simulink model "Manoel_05"  (R2018a)
settings: Solver=VariableStepAuto  StartTime=0.0  StopTime=10.0  RelTol=1e-3
values from neighbouring files (symbols this model uses):
  A = [-4.5 0; 1 -0.2]    [manoel_outubro2.m]    (also in pre6_teste.m; pre_lab5.m; pre_lab6.m; pre_pedro.m = [-5.5 0; 1 -8.40])
  atraso = stt    [manoel_outubro2.m]    (also in naao_roda.m = infor.SettlingTime; pre6_teste.m = infor.SettlingTime; pre_lab3.m = infor.SettlingTime; pre_lab3_lab.m = infor.SettlingTime)
  B = [21.6; 0]    [manoel_outubro2.m]    (also in pre6_teste.m; pre_lab5.m = [18; 0]; pre_lab6.m = [b0; 0]; pre_pedro.m = [462; 0])
  ganho = 0.01027*infor.SettlingMax    [manoel_outubro2.m]    (also in naao_roda.m; pre6_teste.m; pre_lab3.m; pre_lab3_lab.m)
  K = place(Ad, Bd, polos)    [pre6_teste.m]    (also in pre_lab5.m; pre_pedro.m = place(F, H, Dinamica))
  Kpf = 1.0436    [pre_lab3.m]    (also in pre_lab3_lab.m; pre_lab4.m; pre_pedro.m = 1/dcgain(EE))
  R0 = round(r0,1)    [naao_roda.m]    (also in pre6_teste.m; pre_lab3.m; pre_lab3_lab.m; pre_lab4.m)
  T0 = round(t0,3)    [naao_roda.m]    (also in pre6_teste.m = 0.063; pre_lab3.m; pre_lab3_2.m = 0.0640576; pre_lab3_lab.m)
undefined symbols (not defined in the file or in its folder): Ad, Bd
settings Model: Creator=joaovitor  LastModifiedBy=joaovitor

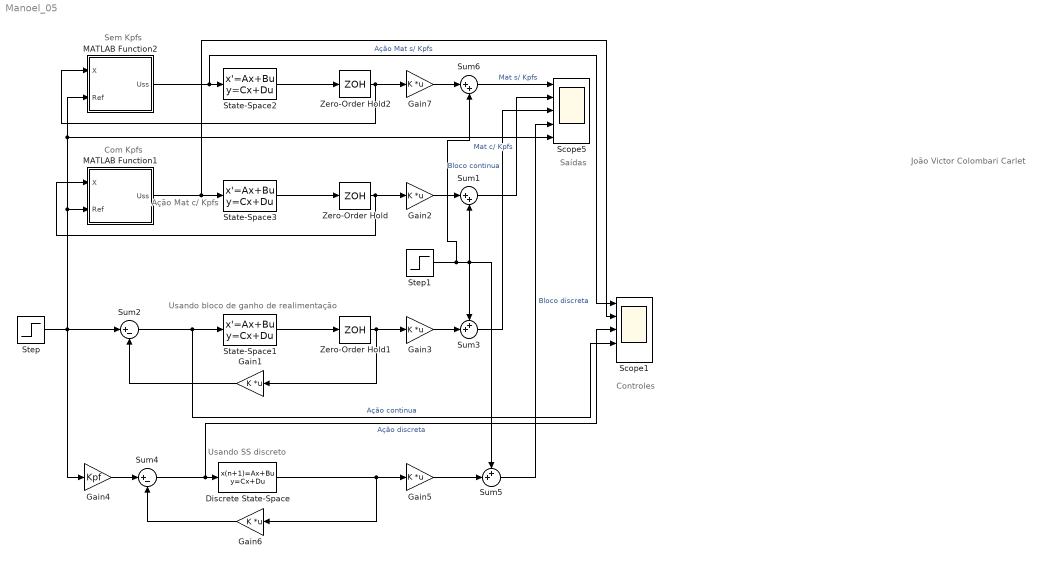
== system Manoel_05 ==
  note: Ação Mat c/ Kpfs
  note: Controles
  note: Saídas
  note: João Victor Colombari Carlet
  note: Usando SS discreto
  note: Usando bloco de ganho de realimentação
  note: Com Kpfs
  note: Sem Kpfs
  Discrete State-Space : DiscreteStateSpace  A=Ad  B=Bd  C=eye(2,2)  D=[0;0]  SampleTime=T0
  Gain{1..3,5..7} (6 alike) : Gain  Gain=K  Multiplication=Matrix(K*u)
  Gain4 : Gain  Gain=Kpf
  MATLAB Function1 : MATLAB Function  TreatAsAtomicUnit=on
  MATLAB Function2 : MATLAB Function  TreatAsAtomicUnit=on
  Scope1 : Scope  NumInputPorts=5
  Scope5 : Scope  NumInputPorts=5
  State-Space1 : StateSpace  A=A  B=B  C=[1 0; 0 1]  D=[0; 0]  InitialCondition=0
  State-Space2 : StateSpace  A=A  B=B  C=[1 0; 0 1]  D=[0; 0]  InitialCondition=0
  State-Space3 : StateSpace  A=A  B=B  C=[1 0; 0 1]  D=[0; 0]  InitialCondition=0
  Step : Step  Time=0  After=R0  SampleTime=0
  Step1 : Step  Time=5*atraso  After=100*ganho  SampleTime=0
  Sum1 : Sum  Inputs=|++
  Sum2 : Sum  Inputs=|+-
  Sum3 : Sum  Inputs=++|
  Sum4 : Sum  Inputs=|+-
  Sum5 : Sum  Inputs=++|
  Sum6 : Sum  Inputs=|++
  Zero-Order Hold : ZeroOrderHold  SampleTime=T0
  Zero-Order Hold1 : ZeroOrderHold  SampleTime=T0
  Zero-Order Hold2 : ZeroOrderHold  SampleTime=T0
  wires:
  MATLAB Function1/1(Uss) -> State-Space3/1, Scope1/2
  State-Space3/1 -> Zero-Order Hold/1
  Zero-Order Hold/1 -> Gain2/1, MATLAB Function1/1(X)
  Step/1 -> Gain4/1, Sum2/1, MATLAB Function1/2(Ref), MATLAB Function2/2(Ref), Scope5/5
  Gain2/1 -> Sum1/1
  Sum2/1 -> State-Space1/1, Scope1/4  "Ação continua"
  State-Space1/1 -> Zero-Order Hold1/1
  Zero-Order Hold1/1 -> Gain1/1, Gain3/1
  Gain3/1 -> Sum3/2
  Step1/1 -> Sum6/2, Sum1/2, Sum3/1, Sum5/1
  Gain1/1 -> Sum2/2
  Gain4/1 -> Sum4/1
  Sum4/1 -> Scope1/3, Discrete State-Space/1  "Ação discreta"
  Gain6/1 -> Sum4/2
  Discrete State-Space/1 -> Gain6/1, Gain5/1
  Gain5/1 -> Sum5/2
  MATLAB Function2/1(Uss) -> Scope1/1, State-Space2/1  "Ação Mat s/ Kpfs"
  State-Space2/1 -> Zero-Order Hold2/1
  Zero-Order Hold2/1 -> MATLAB Function2/1(X), Gain7/1
  Gain7/1 -> Sum6/1
  Sum6/1 -> Scope5/1  "Mat s/ Kpfs"
  Sum1/1 -> Scope5/2  "Mat c/ Kpfs"
  Sum3/1 -> Scope5/3  "Bloco continua"
  Sum5/1 -> Scope5/4  "Bloco discreta"

== matlab function Manoel_05/MATLAB Function1 ==
  data: X input; K parameter; Kpf parameter; Uss output; Ref input
function Uss = fcn(X, K, Kpf, Ref)

Uss= Ref*Kpf-K*X;

== matlab function Manoel_05/MATLAB Function2 ==
  data: X input; K parameter; Kpf parameter; Uss output; Ref input
function Uss = fcn(X, K, Kpf, Ref)

Uss= Ref-K*X;
